simulink subsystem "JacobianX_3DoF"  (R2024b)
settings: Solver=VariableStepAuto  StartTime=0.0  StopTime=10.0  RelTol=1e-3
undefined symbols (not defined in the file or in its folder): com_error, inertia_error, mass_error, vehicle
settings Model: Creator=thatf  LastModifiedBy=thatf

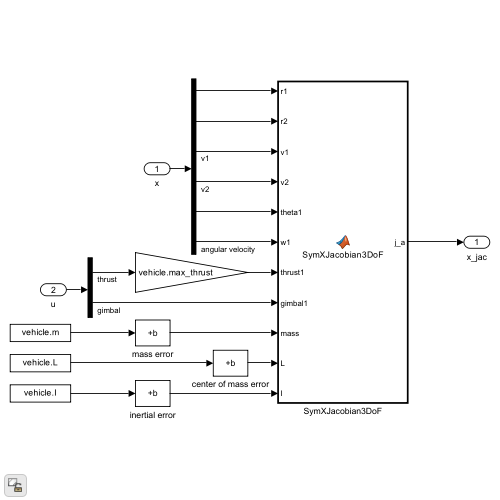
[thumbnail: Simulink's stored preview of the top-level diagram]
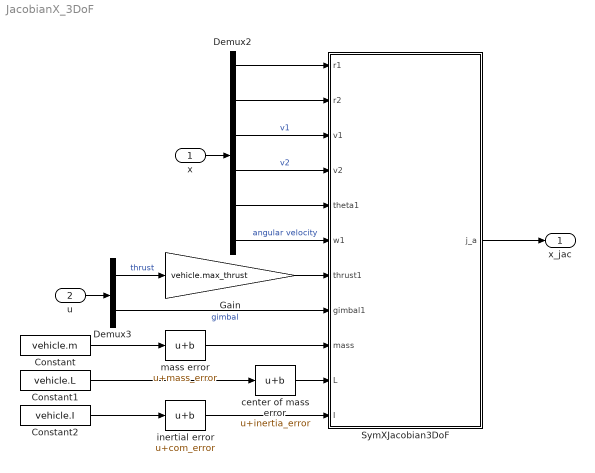
== system JacobianX_3DoF ==
  x : Inport
  u : Inport  Port=2
  Constant : Constant  Value=vehicle.m
  Constant1 : Constant  Value=vehicle.L
  Constant2 : Constant  Value=vehicle.I
  Demux2 : Demux  Outputs=6
  Demux3 : Demux  Outputs=2
  Gain : Gain  Gain=vehicle.max_thrust
  SymXJacobian3DoF : MATLAB Function  TreatAsAtomicUnit=on
  center of mass error : Bias  Bias=inertia_error  SaturateOnIntegerOverflow=off
  inertial error : Bias  Bias=com_error  SaturateOnIntegerOverflow=off
  mass error : Bias  Bias=mass_error  SaturateOnIntegerOverflow=off
  x_jac : Outport
  wires:
  u/1 -> Demux3/1
  x/1 -> Demux2/1
  Demux2/1 -> SymXJacobian3DoF/1(r1)
  Demux2/2 -> SymXJacobian3DoF/2(r2)
  Demux2/3 -> SymXJacobian3DoF/3(v1)  "v1"
  Demux2/4 -> SymXJacobian3DoF/4(v2)  "v2"
  Demux2/5 -> SymXJacobian3DoF/5(theta1)
  Demux2/6 -> SymXJacobian3DoF/6(w1)  "angular velocity"
  Demux3/2 -> SymXJacobian3DoF/8(gimbal1)  "gimbal"
  Constant1/1 -> center of mass error/1
  Constant2/1 -> inertial error/1
  SymXJacobian3DoF/1(j_a) -> x_jac/1
  Gain/1 -> SymXJacobian3DoF/7(thrust1)
  Demux3/1 -> Gain/1  "thrust"
  mass error/1 -> SymXJacobian3DoF/9(mass)
  Constant/1 -> mass error/1
  center of mass error/1 -> SymXJacobian3DoF/10(L)
  inertial error/1 -> SymXJacobian3DoF/11(I)

== matlab function JacobianX_3DoF/SymXJacobian3DoF ==
  data: r1 input; j_a output; r2 input; v1 input; v2 input; theta1 input; w1 input; thrust1 input; gimbal1 input; mass input; L input; I input
function j_a = SymXJacobian3DoF(r1,r2,v1,v2,theta1,w1,thrust1,gimbal1,mass,L,I)
%#codegen

%    This function was generated by the Symbolic Math Toolbox version 24.2.
%    25-Nov-2024 00:53:43

% r1 = complex(r1);  % if required to enforce complex operations
% r2 = complex(r2);  % if required to enforce complex operations
% v1 = complex(v1);  % if required to enforce complex operations
% v2 = complex(v2);  % if required to enforce complex operations
% theta1 = complex(theta1);  % if required to enforce complex operations
% w1 = complex(w1);  % if required to enforce complex operations
% thrust1 = complex(thrust1);  % if required to enforce complex operations
% gimbal1 = complex(gimbal1);  % if required to enforce complex operations
% mass = complex(mass);  % if required to enforce complex operations
% L = complex(L);  % if required to enforce complex operations
% I = complex(I);  % if required to enforce complex operations
t2 = gimbal1+theta1;
t3 = 1.0./mass;
j_a = reshape([0.0,0.0,0.0,0.0,0.0,0.0,0.0,0.0,0.0,0.0,0.0,0.0,1.0,0.0,0.0,0.0,0.0,0.0,0.0,1.0,0.0,0.0,0.0,0.0,0.0,0.0,-t3.*thrust1.*sin(t2),t3.*thrust1.*cos(t2),0.0,0.0,0.0,0.0,0.0,0.0,1.0,0.0],[6,6]);
end
